simulink model "untitled"  (R2017b)
settings: Solver=VariableStepAuto  StartTime=0.0  StopTime=10.0  RelTol=1e-3
undefined symbols (not defined in the file): Km, Kp, Tm
settings Model: Creator=USER  LastModifiedBy=USER

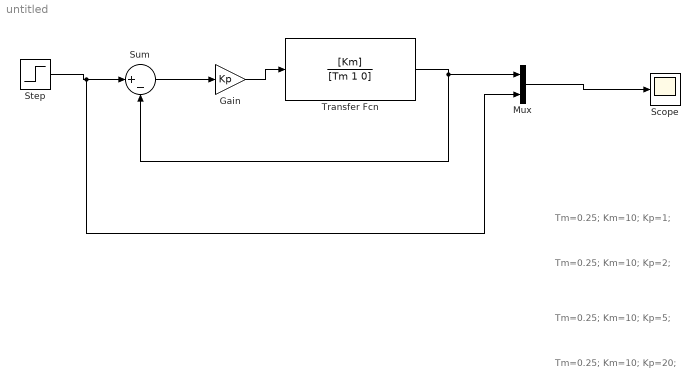
== system untitled ==
  note: Tm=0.25;
      | Km=10;
      | Kp=1;
  note: Tm=0.25;
      | Km=10;
      | Kp=2;
  note: Tm=0.25;
      | Km=10;
      | Kp=5;
  note: Tm=0.25;
      | Km=10;
      | Kp=20;
  Gain : Gain  Gain=Kp
  Mux : Mux  Inputs=2
  Scope : Scope
  Step : Step  Time=0  SampleTime=0
  Sum : Sum  Inputs=|+-
  Transfer Fcn : TransferFcn  Numerator=[Km]  Denominator=[Tm 1 0]
  wires:
  Step/1 -> Mux/2, Sum/1
  Sum/1 -> Gain/1
  Gain/1 -> Transfer Fcn/1
  Transfer Fcn/1 -> Sum/2, Mux/1
  Mux/1 -> Scope/1
